simulink subsystem "actual_adrc_controller"  (R2025a)
settings: Solver=VariableStepAuto  StartTime=0.0  StopTime=10.0  RelTol=1e-3
values from neighbouring files (symbols this model uses):
  dt = constants.dt    [adrc_controller.m]    (also in constants.m = 0.02; dsmc_constraints.m; dsmc_no_constraints.m; hinf_design.m = 0.02)
undefined symbols (not defined in the file or in its folder): constants_struct
settings Model: Creator=johnpye  LastModifiedBy=johnpye

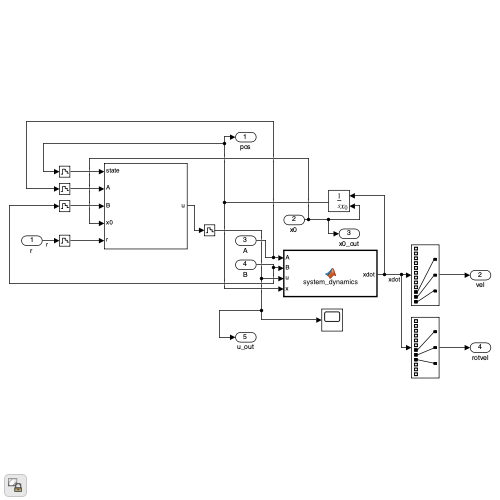
[thumbnail: Simulink's stored preview of the top-level diagram]
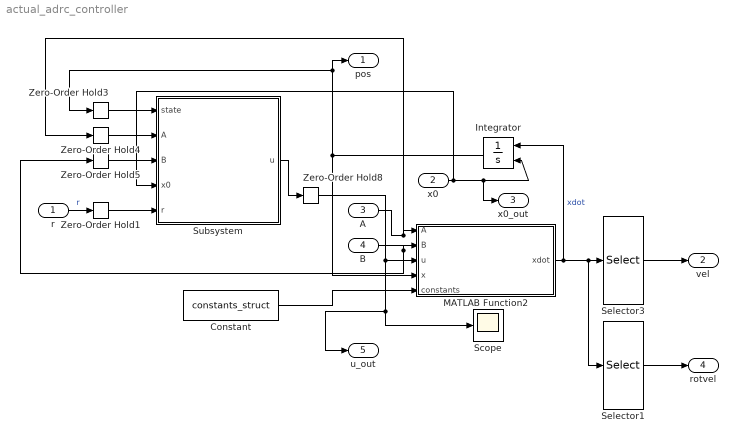
== system actual_adrc_controller ==
  r : Inport
  x0 : Inport  Port=2
  A : Inport  Port=3
  B : Inport  Port=4
  Constant : Constant  Value=constants_struct  OutDataTypeStr=Bus: constants_struct_bus
  Integrator : Integrator  InitialConditionSource=external
  MATLAB Function2 : MATLAB Function  TreatAsAtomicUnit=on
  Scope : Scope
      settings: ActiveDisplayYMinimum=-14.831202203593328  ActiveDisplayYMaximum=20.695169146470946  DataLoggingVariableName=ScopeData8
  Selector1 : Selector  InputPortWidth=12  IndexOptions=Index vector (dialog)  Indices=[7 8 9]  OutputSizes=1
  Selector3 : Selector  InputPortWidth=12  IndexOptions=Index vector (dialog)  Indices=[10 11 12]  OutputSizes=1
  Subsystem : Subsystem
  Zero-Order Hold{1,3..5,8} (5 alike) : ZeroOrderHold  SampleTime=dt
  pos : Outport
  vel : Outport  Port=2
  x0_out : Outport  Port=3
  rotvel : Outport  Port=4
  u_out : Outport  Port=5
  wires:
  Selector3/1 -> vel/1
  x0/1 -> Integrator/2, x0_out/1, Subsystem/4(x0)
  A/1 -> MATLAB Function2/1(A), Zero-Order Hold4/1
  Integrator/1 -> MATLAB Function2/4(x), pos/1, Zero-Order Hold3/1
  B/1 -> Zero-Order Hold5/1, MATLAB Function2/2(B)
  MATLAB Function2/1(xdot) -> Integrator/1, Selector3/1, Selector1/1  "xdot"
  Subsystem/1(u) -> Zero-Order Hold8/1
  Zero-Order Hold1/1 -> Subsystem/5(r)
  Zero-Order Hold3/1 -> Subsystem/1(state)
  Zero-Order Hold4/1 -> Subsystem/2(A)
  Zero-Order Hold5/1 -> Subsystem/3(B)
  Zero-Order Hold8/1 -> MATLAB Function2/3(u), u_out/1, Scope/1
  r/1 -> Zero-Order Hold1/1  "r"
  Selector1/1 -> rotvel/1
  Constant/1 -> MATLAB Function2/5(constants)

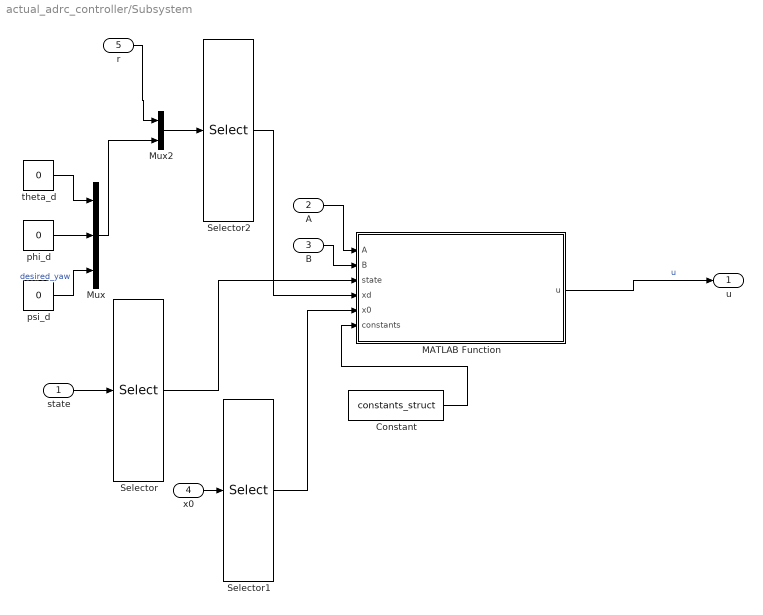
== system actual_adrc_controller/Subsystem ==
  state : Inport
  A : Inport  Port=2
  B : Inport  Port=3
  x0 : Inport  Port=4
  r : Inport  Port=5
  Constant : Constant  Value=constants_struct  OutDataTypeStr=Bus: constants_struct_bus
  MATLAB Function : MATLAB Function  TreatAsAtomicUnit=on
  Mux : Mux  Inputs=3
  Mux2 : Mux  Inputs=2
  Selector : Selector  InputPortWidth=12  IndexOptions=Index vector (dialog)  Indices=[10 11 12 8 7 9 ]  OutputSizes=1
  Selector1 : Selector  InputPortWidth=12  IndexOptions=Index vector (dialog)  Indices=[10 11 12 8 7 9 ]  OutputSizes=1
  Selector2 : Selector  InputPortWidth=6  IndexOptions=Index vector (dialog)  Indices=[1 2 3 5 4 6]  OutputSizes=1
  phi_d : Constant  Value=0
  psi_d : Constant  Value=0
  theta_d : Constant  Value=0
  u : Outport
  wires:
  Constant/1 -> MATLAB Function/6(constants)
  Selector2/1 -> MATLAB Function/4(xd)
  Selector1/1 -> MATLAB Function/5(x0)
  Selector/1 -> MATLAB Function/3(state)
  state/1 -> Selector/1
  theta_d/1 -> Mux/1
  x0/1 -> Selector1/1
  Mux2/1 -> Selector2/1
  r/1 -> Mux2/1
  psi_d/1 -> Mux/3  "desired_yaw"
  B/1 -> MATLAB Function/2(B)
  Mux/1 -> Mux2/2
  phi_d/1 -> Mux/2
  A/1 -> MATLAB Function/1(A)
  MATLAB Function/1(u) -> u/1  "u"

== matlab function actual_adrc_controller/MATLAB Function2 ==
  data: A input; B input; u input; x input; xdot output; constants input
function xdot = func(A, B, u, x, constants)
xdot = system_dynamics(A, B, u, x, constants);

== matlab function actual_adrc_controller/Subsystem/MATLAB Function ==
  data: A input; B input; state input; u output; xd input size=[6; 1]; x0 input; constants input
function u = MATLAB_Function(A, B, state, xd, x0, constants)
u = adrc_controller(A, B, state, xd, x0, constants);
